simulink model "Four_working_Controllers_with_gains"  (R2014b)
settings: Solver=ode45  StartTime=0.0  StopTime=30  FixedStep=0.01  RelTol=1e-3
values from neighbouring files (symbols this model uses):
  A1 = kp/kd    [init.m]
  B1 = kd    (= 0)    [init.m]
  B2 = kd    (= 0)    [init.m]
  controller = 1    [init.m]
  d = 0.06    [init.m]
  g0 = -9.81    [init.m]
  G1 = kp    (= 0)    [init.m]
  G2 = kd    (= 0)    [init.m]
  I = 0.004    [init.m]
  Im = 0.0075    [init.m]
  k = 4.0    (= 4)    [init.m]
  m = 0.03    [init.m]
  q_init = 1.5    [init.m]
  th_init = 1.5    [init.m]
settings Model: Creator=User  LastModifiedBy=User

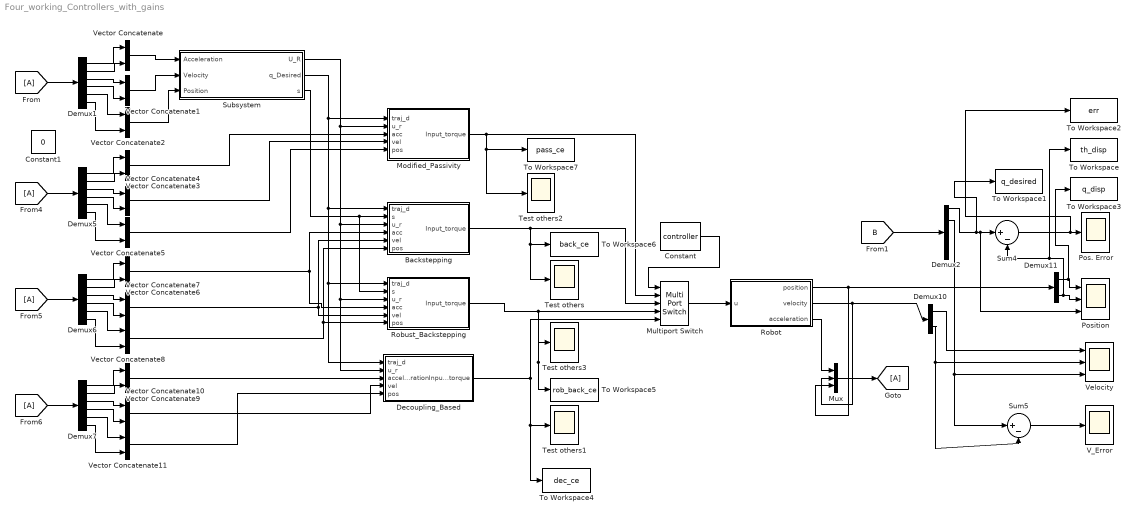
== system Four_working_Controllers_with_gains ==
  Backstepping : Subsystem
  Constant : Constant  Value=controller
  Constant1 : Constant  Value=0
  "Decoupling_Based " : Subsystem
  Demux{1,5..7} (4 alike) : Demux  Outputs=6
  Demux10 : Demux  Outputs=2
  Demux11 : Demux  Outputs=2
  Demux2 : Demux  Outputs=5
  Modified_Passivity : Subsystem
  Multiport Switch : MultiPortSwitch  DataPortOrder=Specify indices  DataPortIndices={1,2,3,4}
  Mux : Mux  Inputs=3
  Pos. Error : Scope
      settings: ShowLegends=on  YMin=-0.3  YMax=0.1  SaveName=ScopeData15
  Position : Scope  NumInputPorts=3
      settings: ShowLegends=on  YMin=-1~-1~-1  YMax=1.5~2~1  SaveName=ScopeData16
  Robot : Subsystem
  Robust_Backstepping : Subsystem
  Subsystem : Subsystem
  Sum4 : Sum  Inputs=|+-
  Sum5 : Sum  Inputs=|+-
  Test others{,1..3} (4 alike) : Scope
      Test others settings: ShowLegends=on  YMin=-0.03  YMax=0.04
      Test others1 settings: ShowLegends=on  YMin=-0.25  YMax=0.1
      Test others2 settings: ShowLegends=on  YMin=-0.5  YMax=0.5  SaveName=ScopeData2
      Test others3 settings: ShowLegends=on  YMin=-0.04  YMax=0.04  SaveName=ScopeData3
  To Workspace : ToWorkspace  VariableName=th_disp  SaveFormat=Timeseries  SampleTime=-1
  To Workspace1 : ToWorkspace  VariableName=q_desired  SaveFormat=Timeseries  SampleTime=-1
  To Workspace2 : ToWorkspace  VariableName=err  SaveFormat=Timeseries  SampleTime=-1
      settings: Save2DSignal=2-D array (concatenate along first dimension)
  To Workspace3 : ToWorkspace  VariableName=q_disp  SaveFormat=Timeseries  SampleTime=-1
  To Workspace4 : ToWorkspace  VariableName=dec_ce  SaveFormat=Timeseries  SampleTime=-1
      settings: Save2DSignal=2-D array (concatenate along first dimension)
  To Workspace5 : ToWorkspace  VariableName=rob_back_ce  SaveFormat=Timeseries  SampleTime=-1
      settings: Save2DSignal=2-D array (concatenate along first dimension)
  To Workspace6 : ToWorkspace  VariableName=back_ce  SaveFormat=Timeseries  SampleTime=-1
      settings: Save2DSignal=2-D array (concatenate along first dimension)
  To Workspace7 : ToWorkspace  VariableName=pass_ce  SaveFormat=Timeseries  SampleTime=-1
      settings: Save2DSignal=2-D array (concatenate along first dimension)
  V_Error : Scope
      settings: ShowLegends=on  YMin=-0.8  YMax=0.8  SaveName=ScopeData20
  Vector Concatenate{,1..11} (12 alike) : Concatenate
  Velocity : Scope  NumInputPorts=3
      settings: YMin=-5~-5~-5  YMax=5~5~5  SaveName=ScopeData21
  wires:
  Backstepping/1(Input_torque) -> Multiport Switch/3, Test others/1, To Workspace6/1
  "Decoupling_Based "/1(Input_torque) -> Multiport Switch/5, To Workspace4/1, Test others1/1
  Modified_Passivity/1(Input_torque) -> Test others2/1, To Workspace7/1, Multiport Switch/2
  Constant/1 -> Multiport Switch/1
  Subsystem/2(q_Desired) -> Robust_Backstepping/1("traj_d "), "Decoupling_Based "/1("traj_d "), Backstepping/1("traj_d "), Modified_Passivity/1("traj_d ")
  Demux10/1 -> Velocity/1
  Robot/2(velocity) -> Mux/2, Demux10/1
  Demux11/2 -> Sum4/2, To Workspace/1, Position/2
  Demux11/1 -> Position/1, To Workspace3/1
  Sum5/1 -> V_Error/1
  Demux10/2 -> Sum5/2, Velocity/2
  Multiport Switch/1 -> Robot/1("u ")
  Subsystem/3(s) -> Robust_Backstepping/2(s), Backstepping/2(s)
  Subsystem/1(U_R) -> Modified_Passivity/2(u_r), Backstepping/3(u_r), Robust_Backstepping/3(u_r), "Decoupling_Based "/2(u_r)
  Mux/1 -> [A]
  Robot/3(acceleration) -> Mux/1
  Robot/1(position) -> Mux/3, Demux11/1
  [A] -> Demux1/1
  Demux1/1 -> Vector Concatenate/1
  Demux1/2 -> Vector Concatenate/2
  Demux1/3 -> Vector Concatenate1/1
  Demux1/4 -> Vector Concatenate1/2
  Demux1/5 -> Vector Concatenate2/1
  Demux1/6 -> Vector Concatenate2/2
  Vector Concatenate/1 -> Subsystem/1(Acceleration)
  Vector Concatenate1/1 -> Subsystem/2(Velocity)
  Vector Concatenate2/1 -> Subsystem/3(Position)
  [A] -> Demux5/1
  Demux5/1 -> Vector Concatenate3/1
  Demux5/2 -> Vector Concatenate3/2
  Demux5/3 -> Vector Concatenate4/1
  Demux5/4 -> Vector Concatenate4/2
  Demux5/5 -> Vector Concatenate5/1
  Demux5/6 -> Vector Concatenate5/2
  Vector Concatenate3/1 -> Modified_Passivity/3(acc)
  Vector Concatenate4/1 -> Modified_Passivity/4(vel)
  Vector Concatenate5/1 -> Modified_Passivity/5(pos)
  [A] -> Demux6/1
  Demux6/1 -> Vector Concatenate6/1
  Demux6/2 -> Vector Concatenate6/2
  Demux6/3 -> Vector Concatenate7/1
  Demux6/4 -> Vector Concatenate7/2
  Demux6/5 -> Vector Concatenate8/1
  Demux6/6 -> Vector Concatenate8/2
  Vector Concatenate6/1 -> Robust_Backstepping/4(acc), Backstepping/4(acc)
  Vector Concatenate7/1 -> Robust_Backstepping/5(vel), Backstepping/5(vel)
  Vector Concatenate8/1 -> Robust_Backstepping/6(pos), Backstepping/6(pos)
  [A] -> Demux7/1
  Demux7/1 -> Vector Concatenate9/1
  Demux7/2 -> Vector Concatenate9/2
  Demux7/3 -> Vector Concatenate10/1
  Demux7/4 -> Vector Concatenate10/2
  Demux7/5 -> Vector Concatenate11/1
  Demux7/6 -> Vector Concatenate11/2
  Vector Concatenate9/1 -> "Decoupling_Based "/3(acceleration)
  Vector Concatenate10/1 -> "Decoupling_Based "/4(vel)
  Vector Concatenate11/1 -> "Decoupling_Based "/5(pos)
  [B] -> Demux2/1
  Demux2/1 -> To Workspace1/1, Position/3, Sum4/1
  Demux2/2 -> Velocity/3, Sum5/1
  Robust_Backstepping/1(Input_torque) -> Multiport Switch/4, To Workspace5/1, Test others3/1
  Sum4/1 -> To Workspace2/1, Pos. Error/1

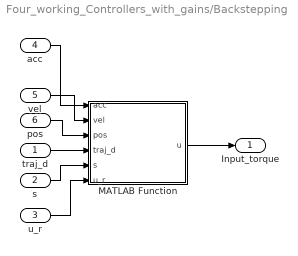
== system Four_working_Controllers_with_gains/Backstepping ==
  "traj_d " : Inport
  s : Inport  Port=2
  u_r : Inport  Port=3
  acc : Inport  Port=4
  vel : Inport  Port=5
  pos : Inport  Port=6
  MATLAB Function : MATLAB Function  TreatAsAtomicUnit=on
  Input_torque : Outport
  wires:
  pos/1 -> MATLAB Function/3(pos)
  vel/1 -> MATLAB Function/2(vel)
  "traj_d "/1 -> MATLAB Function/4(traj_d)
  MATLAB Function/1(u) -> Input_torque/1
  u_r/1 -> MATLAB Function/6(u_r)
  acc/1 -> MATLAB Function/1(acc)
  s/1 -> MATLAB Function/5(s)

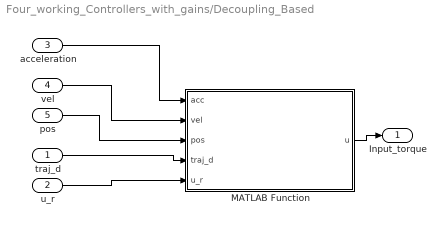
== system Four_working_Controllers_with_gains/Decoupling_Based  ==
  "traj_d " : Inport
  u_r : Inport  Port=2
  acceleration : Inport  Port=3
  vel : Inport  Port=4
  pos : Inport  Port=5
  MATLAB Function : MATLAB Function  TreatAsAtomicUnit=on
  Input_torque : Outport
  wires:
  "traj_d "/1 -> MATLAB Function/4(traj_d)
  MATLAB Function/1(u) -> Input_torque/1
  acceleration/1 -> MATLAB Function/1(acc)
  u_r/1 -> MATLAB Function/5(u_r)
  vel/1 -> MATLAB Function/2(vel)
  pos/1 -> MATLAB Function/3(pos)

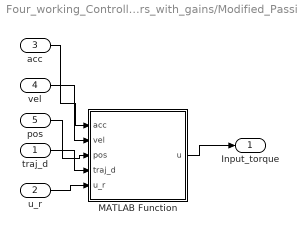
== system Four_working_Controllers_with_gains/Modified_Passivity ==
  "traj_d " : Inport
  u_r : Inport  Port=2
  acc : Inport  Port=3
  vel : Inport  Port=4
  pos : Inport  Port=5
  MATLAB Function : MATLAB Function  TreatAsAtomicUnit=on
  Input_torque : Outport
  wires:
  pos/1 -> MATLAB Function/3(pos)
  vel/1 -> MATLAB Function/2(vel)
  "traj_d "/1 -> MATLAB Function/4(traj_d)
  MATLAB Function/1(u) -> Input_torque/1
  u_r/1 -> MATLAB Function/5(u_r)
  acc/1 -> MATLAB Function/1(acc)

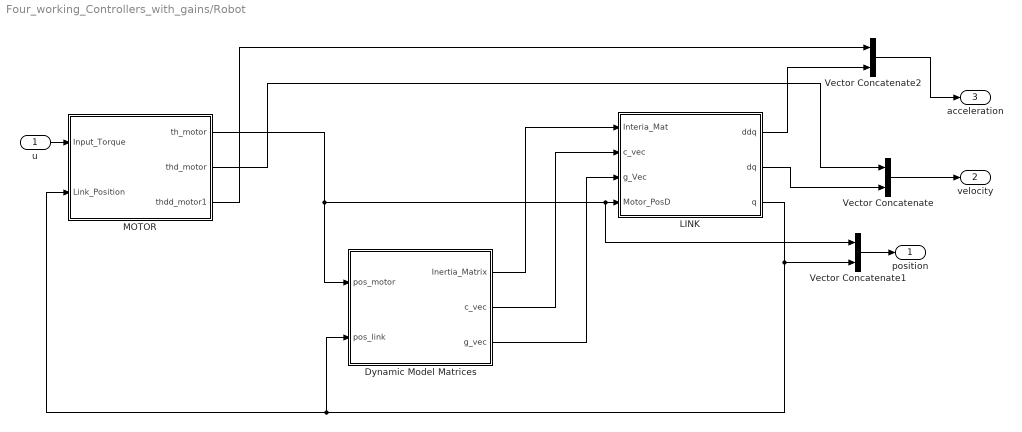
== system Four_working_Controllers_with_gains/Robot ==
  "u " : Inport
  Dynamic Model Matrices : Subsystem
  LINK : Subsystem
  MOTOR : Subsystem
  Vector Concatenate : Concatenate
  Vector Concatenate1 : Concatenate
  Vector Concatenate2 : Concatenate
  position : Outport
  velocity : Outport  Port=2
  acceleration : Outport  Port=3
  wires:
  "u "/1 -> MOTOR/1(Input_Torque)
  Dynamic Model Matrices/1(Inertia_Matrix) -> LINK/1(Interia_Mat)
  Dynamic Model Matrices/2(c_vec) -> LINK/2(c_vec)
  Dynamic Model Matrices/3(g_vec) -> LINK/3(g_Vec)
  MOTOR/1(th_motor) -> Vector Concatenate1/1, LINK/4(Motor_PosD), Dynamic Model Matrices/1(pos_motor)
  LINK/3(q) -> Vector Concatenate1/2, Dynamic Model Matrices/2(pos_link), MOTOR/2(Link_Position)
  MOTOR/2(thd_motor) -> Vector Concatenate/1
  LINK/2(dq) -> Vector Concatenate/2
  Vector Concatenate/1 -> velocity/1
  Vector Concatenate1/1 -> position/1
  Vector Concatenate2/1 -> acceleration/1
  MOTOR/3(thdd_motor1) -> Vector Concatenate2/1
  LINK/1(ddq) -> Vector Concatenate2/2

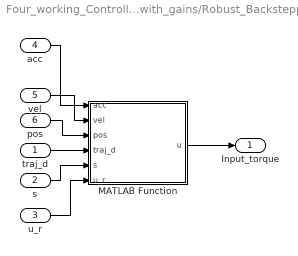
== system Four_working_Controllers_with_gains/Robust_Backstepping ==
  "traj_d " : Inport
  s : Inport  Port=2
  u_r : Inport  Port=3
  acc : Inport  Port=4
  vel : Inport  Port=5
  pos : Inport  Port=6
  MATLAB Function : MATLAB Function  TreatAsAtomicUnit=on
  Input_torque : Outport
  wires:
  s/1 -> MATLAB Function/5(s)
  acc/1 -> MATLAB Function/1(acc)
  u_r/1 -> MATLAB Function/6(u_r)
  MATLAB Function/1(u) -> Input_torque/1
  "traj_d "/1 -> MATLAB Function/4(traj_d)
  vel/1 -> MATLAB Function/2(vel)
  pos/1 -> MATLAB Function/3(pos)

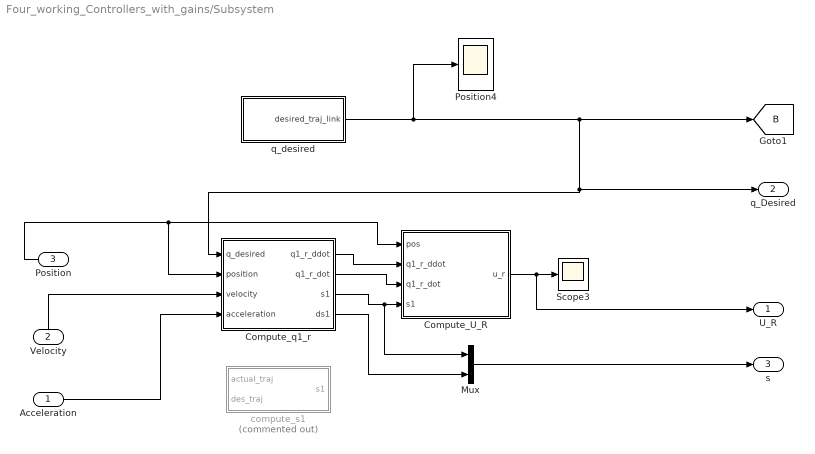
== system Four_working_Controllers_with_gains/Subsystem ==
  Acceleration : Inport
  Velocity : Inport  Port=2
  Position : Inport  Port=3
  Compute_U_R : Subsystem
  Compute_q1_r : Subsystem
  Mux : Mux  Inputs=2
  Position4 : Scope
      settings: ShowLegends=on  YMin=-9e+115  YMax=1e+115  SaveName=ScopeData17
  Scope3 : Scope
      settings: YMin=-1.75193  YMax=1.87977  SaveName=ScopeData19
  compute_s1 : Subsystem  Commented=on
  q_desired : Subsystem
  U_R : Outport
  q_Desired : Outport  Port=2
  s : Outport  Port=3
  tag scope: B=global
  wires:
  q_desired/1(desired_traj_link) -> Position4/1, [B], q_Desired/1, Compute_q1_r/1(q_desired)
  Compute_q1_r/1(q1_r_ddot) -> Compute_U_R/2(q1_r_ddot)
  Compute_q1_r/2(q1_r_dot) -> Compute_U_R/3(q1_r_dot)
  Compute_U_R/1(u_r) -> U_R/1, Scope3/1
  Position/1 -> Compute_U_R/1(pos), Compute_q1_r/2(position)
  Velocity/1 -> Compute_q1_r/3(velocity)
  Acceleration/1 -> Compute_q1_r/4(acceleration)
  Compute_q1_r/4(ds1) -> Mux/2
  Compute_q1_r/3(s1) -> Mux/1, Compute_U_R/4(s1)
  Mux/1 -> s/1

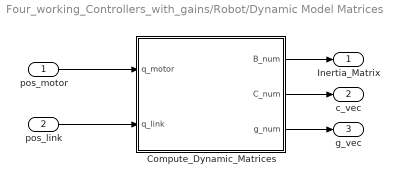
== system Four_working_Controllers_with_gains/Robot/Dynamic Model Matrices ==
  pos_motor : Inport
  pos_link : Inport  Port=2
  Compute_Dynamic_Matrices : MATLAB Function  TreatAsAtomicUnit=on
  Inertia_Matrix : Outport
  c_vec : Outport  Port=2
  g_vec : Outport  Port=3
  wires:
  Compute_Dynamic_Matrices/1(B_num) -> Inertia_Matrix/1
  Compute_Dynamic_Matrices/2(C_num) -> c_vec/1
  Compute_Dynamic_Matrices/3(g_num) -> g_vec/1
  pos_motor/1 -> Compute_Dynamic_Matrices/1(q_motor)
  pos_link/1 -> Compute_Dynamic_Matrices/2(q_link)

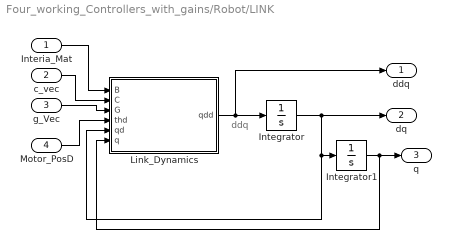
== system Four_working_Controllers_with_gains/Robot/LINK ==
  note: ddq
  Interia_Mat : Inport
  c_vec : Inport  Port=2
  g_Vec : Inport  Port=3
  Motor_PosD : Inport  Port=4
  Integrator : Integrator
  Integrator1 : Integrator  InitialCondition=q_init
  Link_Dynamics : MATLAB Function  TreatAsAtomicUnit=on
  ddq : Outport
  dq : Outport  Port=2
  q : Outport  Port=3
  wires:
  Link_Dynamics/1(qdd) -> ddq/1, Integrator/1
  Integrator/1 -> Link_Dynamics/5(qd), Integrator1/1, dq/1
  Integrator1/1 -> q/1, Link_Dynamics/6(q)
  Motor_PosD/1 -> Link_Dynamics/4(thd)
  Interia_Mat/1 -> Link_Dynamics/1(B)
  c_vec/1 -> Link_Dynamics/2(C)
  g_Vec/1 -> Link_Dynamics/3(G)

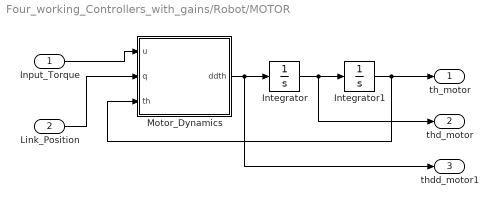
== system Four_working_Controllers_with_gains/Robot/MOTOR ==
  Input_Torque : Inport
  Link_Position : Inport  Port=2
  Integrator : Integrator
  Integrator1 : Integrator  InitialCondition=th_init
  Motor_Dynamics : MATLAB Function  TreatAsAtomicUnit=on
  th_motor : Outport
  thd_motor : Outport  Port=2
  thdd_motor1 : Outport  Port=3
  wires:
  Input_Torque/1 -> Motor_Dynamics/1(u)
  Motor_Dynamics/1(ddth) -> thdd_motor1/1, Integrator/1
  Integrator/1 -> thd_motor/1, Integrator1/1
  Integrator1/1 -> Motor_Dynamics/3(th), th_motor/1
  Link_Position/1 -> Motor_Dynamics/2(q)

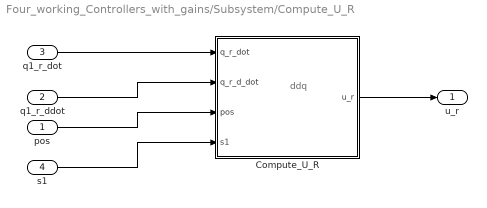
== system Four_working_Controllers_with_gains/Subsystem/Compute_U_R ==
  note: ddq
  pos : Inport
  q1_r_ddot : Inport  Port=2
  q1_r_dot : Inport  Port=3
  s1 : Inport  Port=4
  Compute_U_R : MATLAB Function  TreatAsAtomicUnit=on
  u_r : Outport
  wires:
  Compute_U_R/1(u_r) -> u_r/1
  q1_r_dot/1 -> Compute_U_R/1(q_r_dot)
  q1_r_ddot/1 -> Compute_U_R/2(q_r_d_dot)
  s1/1 -> Compute_U_R/4(s1)
  pos/1 -> Compute_U_R/3(pos)

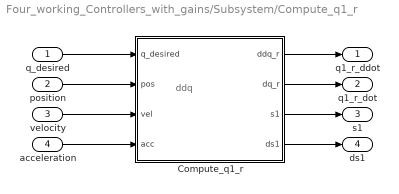
== system Four_working_Controllers_with_gains/Subsystem/Compute_q1_r ==
  note: ddq
  q_desired : Inport
  position : Inport  Port=2
  velocity : Inport  Port=3
  acceleration : Inport  Port=4
  Compute_q1_r : MATLAB Function  TreatAsAtomicUnit=on
  q1_r_ddot : Outport
  q1_r_dot : Outport  Port=2
  s1 : Outport  Port=3
  ds1 : Outport  Port=4
  wires:
  Compute_q1_r/3(s1) -> s1/1
  velocity/1 -> Compute_q1_r/3(vel)
  Compute_q1_r/1(ddq_r) -> q1_r_ddot/1
  Compute_q1_r/2(dq_r) -> q1_r_dot/1
  position/1 -> Compute_q1_r/2(pos)
  q_desired/1 -> Compute_q1_r/1(q_desired)
  acceleration/1 -> Compute_q1_r/4(acc)
  Compute_q1_r/4(ds1) -> ds1/1

== system Four_working_Controllers_with_gains/Subsystem/compute_s1 ==
  actual_traj : Inport
  des_traj : Inport  Port=2
  Integrator : Integrator
  MATLAB Function : MATLAB Function  TreatAsAtomicUnit=on
  Vector Concatenate : Concatenate
  s1 : Outport
  wires:
  MATLAB Function/1(s1_d) -> Vector Concatenate/2, Integrator/1
  Integrator/1 -> Vector Concatenate/1
  Vector Concatenate/1 -> s1/1
  des_traj/1 -> MATLAB Function/1(q_d)
  actual_traj/1 -> MATLAB Function/2(q)

== system Four_working_Controllers_with_gains/Subsystem/q_desired ==
  Clock : Clock
  MATLAB Function : MATLAB Function  TreatAsAtomicUnit=on
  To Workspace : ToWorkspace  VariableName=time  SaveFormat=Timeseries  SampleTime=-1
      settings: Save2DSignal=2-D array (concatenate along first dimension)
  Vector Concatenate : Concatenate  NumInputs=5
  desired_traj_link : Outport
  wires:
  Clock/1 -> To Workspace/1, MATLAB Function/1(t)
  Vector Concatenate/1 -> desired_traj_link/1
  MATLAB Function/1(ddddq_d) -> Vector Concatenate/5
  MATLAB Function/2(dddq_d) -> Vector Concatenate/4
  MATLAB Function/3(ddq_d) -> Vector Concatenate/3
  MATLAB Function/4(dq_d) -> Vector Concatenate/2
  MATLAB Function/5(q_d) -> Vector Concatenate/1

== matlab function Four_working_Controllers_with_gains/Backstepping/MATLAB Function ==
  data: acc input; vel input; pos input; u output; traj_d input; s input; u_r input; k parameter; Im parameter; d parameter; I parameter; m parameter; g0 parameter
function u = fcn(acc,vel, pos, traj_d, s, u_r, k, Im, d, I, m, g0)
th = pos(1);
q = pos(2);

dth = vel(1);
dq = vel(2);

ddth = acc(1);
ddq = acc(2);

ds1 = s(2);
s1 = s(1);

D = I + (m*d^2);
th_d = (1 / k) * u_r + q;

dg = k * (dq - dth) + m * g0 * d * cos(q) * dq;
dth_d = (1 / k) * ((D * traj_d(4)) + dg) + dq;

ddg = (-d*g0*m*sin(q) * dq) + (k * (ddq - ddth) + m * g0 * d * cos(q) * ddq);
ddth_d = (1 / k) * ((D * traj_d(5)) + ddg) + ddq;

e = th-th_d;
de = dth-dth_d;

u = Im * ( ddth_d - 2*de - 2*e - (k * (ds1 + s1))  ) + ( th - q );

== matlab function Four_working_Controllers_with_gains/Robust_Backstepping/MATLAB Function ==
  data: acc input; vel input; pos input; u output; traj_d input; s input; u_r input; k parameter; Im parameter; d parameter; I parameter; m parameter; g0 parameter
function u = fcn(acc,vel, pos, traj_d, s, u_r, k, Im, d, I, m, g0)
th = pos(1);
q = pos(2);

dth = vel(1);
dq = vel(2);

ddth = acc(1);
ddq = acc(2);

ds1 = s(2);
s1 = s(1);

D = I + (m*d^2);
th_d = (1 / k) * u_r + q;

dg = k * (dq - dth) + m * g0 * d * cos(q) * dq;
dth_d = (1 / k) * ((D * traj_d(4)) + dg) + dq;

ddg = (-d*g0*m*sin(q) * dq) + (k * (ddq - ddth) + m * g0 * d * cos(q) * ddq);
ddth_d = (1 / k) * ((D * traj_d(5)) + ddg) + ddq;

e = th-th_d;
de = dth-dth_d;

u = Im * ( ddth_d - 2*de - 2*e - (k * (ds1 + s1))  ) + ( th - q );

== matlab function Four_working_Controllers_with_gains/Subsystem/compute_s1/MATLAB Function ==
  data: q_d input; q input; s1_d output; A1 parameter
function s1_d = fcn(q_d, q, A1)
ed  = q(1) - q_d(2);
edd = q(2) - q_d(3);
s1_d = edd + A1 * ed;

== matlab function Four_working_Controllers_with_gains/Decoupling_Based /MATLAB Function ==
  data: acc input; vel input; pos input; u output; traj_d input; u_r input; k parameter; Im parameter; G1 parameter; G2 parameter; d parameter; I parameter; m parameter; g0 parameter
function u = fcn(acc, vel, pos, traj_d, u_r, k, Im, G1, G2, d, I, m, g0)
coder.extrinsic('assignin')

th = pos(1);
q = pos(2);

dth = vel(1);
dq = vel(2);

ddth = acc(1);
ddq = acc(2);

D = I + (m*d^2);
th_d = (1 / k) * u_r + q;

dg = k * (dq - dth) + m * g0 * d * cos(q) * dq;
dth_d = (1 / k) * ((D * traj_d(4)) + dg) + dq;

ddg = (-d*g0*m*sin(q) * dq) + (k * (ddq - ddth) + m * g0 * d * cos(q) * ddq);
ddth_d = (1 / k) * ((D * traj_d(5)) + ddg) + ddq;

e = th-th_d;
de = dth-dth_d;

u = k*(th-q) - G1*e - G2*de + Im*ddth_d;

assignin('base','G1',G1)
assignin('base','G2',G2)
% if flag == 0
%     disp('G1 is')
%     disp(G1)
%     disp('G2 is')
%     disp(G2)
%     flag = 1;
% elseif flag == 1
%     disp()
% end
% u = k*(th_d-q) - G1*e - G2*de + Im*ddth_d;
% disp(k*(th_d-q));

== matlab function Four_working_Controllers_with_gains/Subsystem/Compute_U_R/Compute_U_R ==
  data: q_r_dot input; q_r_d_dot input; pos input; u_r output; s1 input; B1 parameter; I parameter; m parameter; g0 parameter; k parameter; d parameter
function u_r = fcn(q_r_dot, q_r_d_dot, pos, s1, B1, I, m, g0, k, d)
coder.extrinsic('assignin')

th = pos(1);
q = pos(2);

D = I + (m*d^2);
c = 0;
g = k*(q - th) + m*g0*d*sin(q);

u_r = (D * q_r_d_dot) + (c * q_r_dot) + (g - (B1 * s1));

assignin('base','B1',B1)
% if flag == 0
%     disp('B1 is')
%     disp(B1)
%     flag = 1;
% elseif flag == 1
%     disp()
% end
% disp('Compute U R')
% disp('ur is')
% disp(u_r)

== matlab function Four_working_Controllers_with_gains/Subsystem/Compute_q1_r/Compute_q1_r ==
  data: q_desired input; pos input; ddq_r output; dq_r output; vel input; acc input; A1 parameter; s1 output; ds1 output
function [ddq_r,dq_r, s1, ds1] = fcn(q_desired, pos, vel, acc, A1)
coder.extrinsic('assignin')

%Real robot parameters
q = pos(2);
dq = vel(2);
ddq = acc(2);


ddq_r = q_desired(3) - (A1 * (dq - q_desired(2)));

dq_r = q_desired(2) - (A1 * (q - q_desired(1)));


% ed  = q(1) - q_d(2);
% edd = q(2) - q_d(3);
% ds1 = edd + A1 * ed;
ds1 = (ddq - q_desired(3)) + ( A1 * (dq - q_desired(2)));
s1 = (dq - q_desired(2)) + ( A1 * (q - q_desired(1)));


assignin('base','A1',A1)
% if flag == 0
%     disp('A1 in Q_R is')
%     disp(A1)
%     flag = 1;
% elseif flag == 1
%     disp()
% end

== matlab function Four_working_Controllers_with_gains/Modified_Passivity/MATLAB Function ==
  data: acc input; vel input; pos input; u output; traj_d input; u_r input; k parameter; Im parameter; d parameter; I parameter; m parameter; g0 parameter; A1 parameter; B2 parameter
function u = fcn(acc,vel, pos, traj_d, u_r, k, Im, d, I, m, g0, A1, B2)
coder.extrinsic('assignin')
th = pos(1);
q = pos(2);

dth = vel(1);
dq = vel(2);

ddth = acc(1);
ddq = acc(2);

D = I + (m*d^2);
th_d = (1 / k) * u_r + q;

dg = k * (dq - dth) + m * g0 * d * cos(q) * dq;
% dth_d = (1 / k) * ((D * traj_d(4)) + dg) + dq;
dth_d = (1 / k) * ((D * traj_d(4)) + dg) + traj_d(2);

ddg = (-d*g0*m*sin(q) * dq) + (k * (ddq - ddth) + m * g0 * d * cos(q) * ddq);
% ddth_d = (1 / k) * ((D * traj_d(5)) + ddg) + ddq;
ddth_d = (1 / k) * ((D * traj_d(5)) + ddg) + traj_d(3);

e = th-th_d;
de = dth-dth_d;

s2 = de + A1 * (e);
ddth_r = ddth_d - A1 * (de);

u = k*(th_d - traj_d(1)) - B2 * s2 + Im*ddth_r;

assignin('base','A1',A1)
assignin('base','B2',B2)
% if flag == 0
%     disp('A1 is')
%     disp(A1)
%     disp('B2 is')
%     disp(B2)
%     flag = 1;
% elseif flag == 1
%     disp()
% end

== matlab function Four_working_Controllers_with_gains/Robot/Dynamic Model Matrices/Compute_Dynamic_Matrices ==
  data: q_motor input size=1,1; q_link input size=1,1; B_num output size=2,2; C_num output size=2,1; g_num output size=2,1; m parameter; d parameter; Im parameter; I parameter; k parameter; g0 parameter
function [B_num, C_num, g_num] = fcn(q_motor, q_link, m, d, Im, I, k, g0)

q = q_link;
th = q_motor;
%dq = vel_link;
%dth = vel_motor;

% disp('***robot inertia matrix***')

B_numeric = [ Im, 0; 0, m*d^2+I];
% disp(B_numeric)
% size(B_numeric)

%disp('*Christoffel matrices*')

%qt=[q;th];
%b1=B(:,1);
%C1=(1/2)*(jacobian(b1,qt)+jacobian(b1,qt).'-diff(B,q));
%b2=B(:,2);
%C2=(1/2)*(jacobian(b2,qt)+jacobian(b2,qt).'-diff(B,th));

%disp('***robot Coriolis and centrifugal term***')


c1 = 0.05;
c2 = 0.05;
c=[c1;c2];
size(c);

% disp('**robot total potential energy**')
% disp('***robot gravity+elasticity term***')

G_numeric = [(th - q)*k; (q - th)*k + d*g0*m*sin(q)]; % my ref is the conventional upward Y-axis
% disp(G_numeric);
% size(G_numeric)


B_num = B_numeric;
C_num = c;
g_num = G_numeric;


%a = sim('Combined_model','SimulationMode','normal');
% b = Combined_model.get('simout')
% assignin('base','b',b);


% set_param('Combined_model','SimulationCommand','pause')
% set_param('Combined_model','SimulationCommand','continue')

== matlab function Four_working_Controllers_with_gains/Robot/LINK/Link_Dynamics ==
  data: B input size=2,2; C input; G input; thd input; qd input; qdd output; q input; k parameter
function qdd = fcn(B, C, G, thd, qd, q, k)
%Real robot parameters
D = B(2,2);
c = C;
g = G;
% I = 7.5;
% C = 2;
% g = q;
qdd = (1/D) * ((k * (thd - q)) - (c(2,1) * qd) - g(2,1));

== matlab function Four_working_Controllers_with_gains/Robot/MOTOR/Motor_Dynamics ==
  data: Im parameter size=1,1; u input size=1,1; q input; th input; ddth output size=1,1; k parameter
function ddth = fcn(Im, u, q, th, k)
%Real robot parameters

% figure
% grid on
% bode(th);
ddth = (1/Im)*(u - (k* (th - q)));

== matlab function Four_working_Controllers_with_gains/Subsystem/q_desired/MATLAB Function ==
  data: t input; ddddq_d output; dddq_d output; ddq_d output; dq_d output; q_d output
function [ddddq_d, dddq_d, ddq_d, dq_d, q_d]  = fcn(t)

ddddq_d = cos(t);
dddq_d = sin(t);
ddq_d = -cos(t);
dq_d = -sin(t);
q_d = cos(t);
